simulink model "cruise_ctrl"  (Simulink 7.0)
settings: Solver=ode45  StartTime=0.0  StopTime=60  MaxStep=0.1  RelTol=1e-3
PreLoadFcn:
  | m = 1000;
  | alpha = [40, 25, 16, 12, 10];
  | Tm = 190;
  | wm = 420;
  | beta = 0.4;
  | Cr = 0.01;
  | rho = 1.3;
  | Cd = 0.32;
  | A = 2.4;
  | g = 9.8;
  | theta = 0;
  | gear = 3;
libraries: simulink x1
settings Model: Creator=Cole Lepine  LastModifiedBy=Cole Lepine

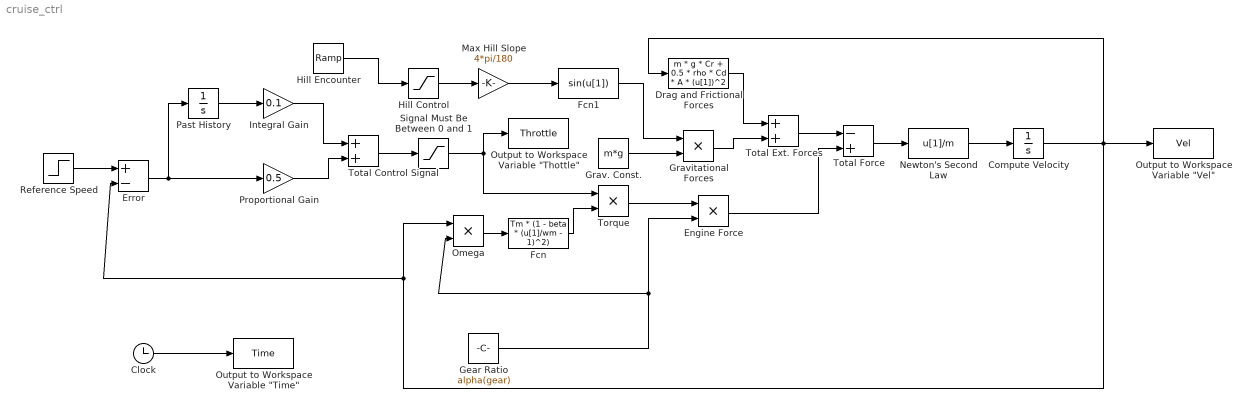
== system cruise_ctrl ==
  Clock : Clock
      settings: Decimation=10
  Compute Velocity : Integrator  InitialCondition=20
  Drag and Frictional Forces : Fcn  Expr=m * g * Cr + 0.5 * rho * Cd * A * (u[1])^2
  Engine Force : Product  Inputs=**  OutDataType=sfix(16)  OutScaling=2^-10
  Error : Sum  Inputs=+-  OutDataType=sfix(16)  OutScaling=2^-10
  Fcn : Fcn  Expr=Tm * (1 - beta * (u[1]/wm - 1)^2)
  Fcn1 : Fcn
  Gear Ratio : Constant  Value=alpha(gear)  OutDataType=sfix(16)  OutScaling=2^0
  Grav. Const. : Constant  Value=m*g  OutDataType=sfix(16)  OutScaling=2^0
  Gravitational Forces : Product  OutDataType=sfix(16)  OutScaling=2^0  RndMeth=Zero
  Hill Control : Saturate  UpperLimit=1  LowerLimit=0  OutDataType=sfix(16)  OutScaling=2^0
  Hill Encounter : simulink/Sources/Ramp  SystemSampleTime=-1  slope=1  start=60  X0=0
  Integral Gain : Gain  Gain=0.1  ParameterDataType=sfix(16)  ParameterScaling=2^0  OutDataType=sfix(16)  OutScaling=2^0
  Max Hill Slope : Gain  Gain=4*pi/180  ParameterDataType=sfix(16)  ParameterScaling=2^0  OutDataType=sfix(16)  OutScaling=2^0
  Newton's Second Law : Fcn  Expr=u[1]/m
  Omega : Product  OutDataType=sfix(16)  OutScaling=2^0  RndMeth=Zero
  "Output to Workspace Variable \"Thottle\"" : ToWorkspace  VariableName=Throttle  SampleTime=-1  SaveFormat=Array
  "Output to Workspace Variable \"Time\"" : ToWorkspace  VariableName=Time  SampleTime=-1  SaveFormat=Array
      settings: Decimation=2
  "Output to Workspace Variable \"Vel\"" : ToWorkspace  VariableName=Vel  SampleTime=-1  SaveFormat=Array
      settings: Decimation=2
  Past History : Integrator  InitialCondition=1
  Proportional Gain : Gain  Gain=0.5  ParameterDataType=sfix(16)  ParameterScaling=2^0  OutDataType=sfix(16)  OutScaling=2^0
  Reference Speed : Step  Time=20  Before=20  After=30  SampleTime=0
  Signal Must Be Between 0 and 1 : Saturate  UpperLimit=1  LowerLimit=0  OutDataType=sfix(16)  OutScaling=2^0
  Torque : Product  OutDataType=sfix(16)  OutScaling=2^0  RndMeth=Zero
  Total Ext. Forces : Sum  OutDataType=sfix(16)  OutScaling=2^-10
  Total Control Signal : Sum  OutDataType=sfix(16)  OutScaling=2^-10
  Total Force : Sum  Inputs=-+  OutDataType=sfix(16)  OutScaling=2^-10
  wires:
  Engine Force/1 -> Total Force/2
  Total Force/1 -> Newton's Second Law/1
  Newton's Second Law/1 -> Compute Velocity/1
  Compute Velocity/1 -> Omega/1, Error/2, "Output to Workspace Variable \"Vel\""/1, Drag and Frictional Forces/1
  Gear Ratio/1 -> Engine Force/2, Omega/2
  Omega/1 -> Fcn/1
  Torque/1 -> Engine Force/1
  Fcn/1 -> Torque/2
  Signal Must Be Between 0 and 1/1 -> Torque/1, "Output to Workspace Variable \"Thottle\""/1
  Reference Speed/1 -> Error/1
  Total Control Signal/1 -> Signal Must Be Between 0 and 1/1
  Proportional Gain/1 -> Total Control Signal/2
  Integral Gain/1 -> Total Control Signal/1
  Error/1 -> Proportional Gain/1, Past History/1
  Past History/1 -> Integral Gain/1
  Clock/1 -> "Output to Workspace Variable \"Time\""/1
  Total Ext. Forces/1 -> Total Force/1
  Drag and Frictional Forces/1 -> Total Ext. Forces/1
  Gravitational Forces/1 -> Total Ext. Forces/2
  Fcn1/1 -> Gravitational Forces/1
  Max Hill Slope/1 -> Fcn1/1
  Grav. Const./1 -> Gravitational Forces/2
  Hill Control/1 -> Max Hill Slope/1
  Hill Encounter/1 -> Hill Control/1
